simulink library "resolveCOM_ul"  (R2018b)
settings: Solver=VariableStepAuto  StartTime=0.0  StopTime=10.0  RelTol=1e-3
settings Model: Creator=MAE-NCSUCORE  LastModifiedBy=MAE-NCSUCORE

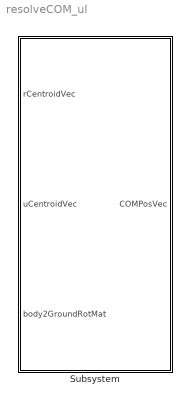
== system resolveCOM_ul ==
  Subsystem : Subsystem  mask{sideDotPosVec_cm=0, botADotPosVec_cm=0, botBDotPosVec_cm=0}

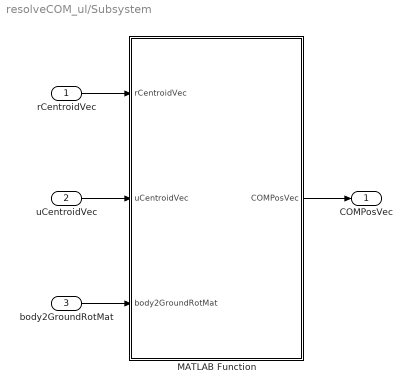
== system resolveCOM_ul/Subsystem ==
  rCentroidVec : Inport
  uCentroidVec : Inport  Port=2
  body2GroundRotMat : Inport  Port=3
  MATLAB Function : MATLAB Function  TreatAsAtomicUnit=on
  COMPosVec : Outport
  wires:
  body2GroundRotMat/1 -> MATLAB Function/3(body2GroundRotMat)
  MATLAB Function/1(COMPosVec) -> COMPosVec/1
  uCentroidVec/1 -> MATLAB Function/2(uCentroidVec)
  rCentroidVec/1 -> MATLAB Function/1(rCentroidVec)

== matlab function resolveCOM_ul/Subsystem/MATLAB Function ==
  data: rCentroidVec input; COMPosVec output; uCentroidVec input; body2GroundRotMat input; sideDotPosVec_cm parameter; botADotPosVec_cm parameter; botBDotPosVec_cm parameter
function COMPosVec  = resolveCOM(rCentroidVec,uCentroidVec,...
    body2GroundRotMat,sideDotPosVec_cm,botADotPosVec_cm,botBDotPosVec_cm)

[COMPosVec] = resolveCOM(rCentroidVec,uCentroidVec,...
    body2GroundRotMat,sideDotPosVec_cm,botADotPosVec_cm,botBDotPosVec_cm);
